simulink model "car_kin_test"  (R2018b)
settings: Solver=FixedStepAuto  StartTime=0.0  StopTime=50  FixedStep=0.05  RelTol=1e-3
libraries: simulink x2, autolibshared x1
settings Model: Creator=le'e'x'  LastModifiedBy=le'e'x'

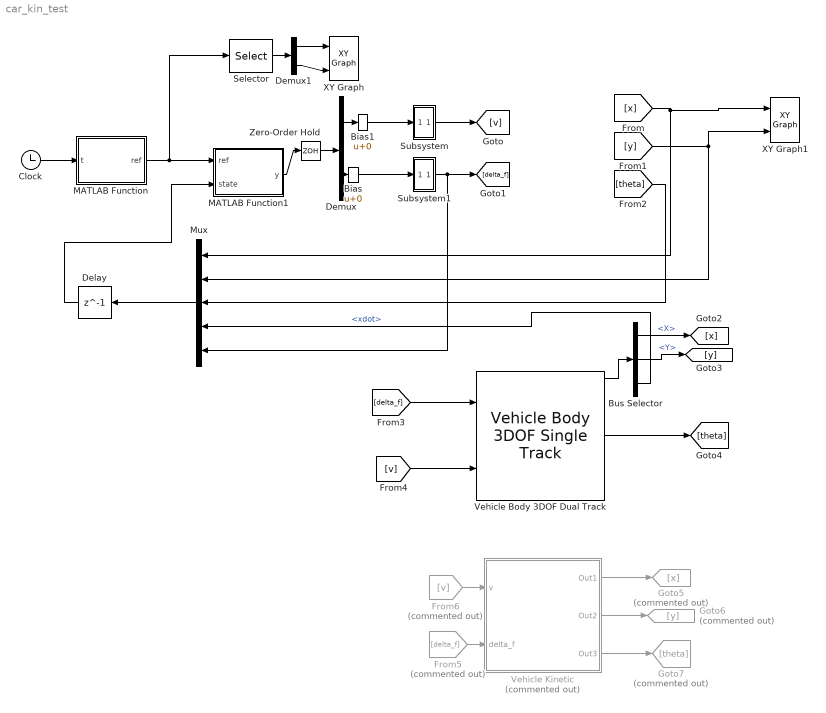
== system car_kin_test ==
  Bias : Bias
  Bias1 : Bias
  Bus Selector : BusSelector  OutputSignals=InertFrm.RearAxl.Disp.X,InertFrm.RearAxl.Disp.Y,BdyFrm.Cg.Vel.xdot
  Clock : Clock
  Delay : Delay  DelayLength=1  InitialCondition=[0 0 0 -0 0]
  Demux : Demux  Outputs=2
  Demux1 : Demux  Outputs=2
  From5 : From  Commented=on  GotoTag=delta_f
  From6 : From  Commented=on  GotoTag=v
  Goto5 : Goto  Commented=on  GotoTag=x
  Goto6 : Goto  Commented=on  GotoTag=y
  Goto7 : Goto  Commented=on  GotoTag=theta
  MATLAB Function : MATLAB Function  TreatAsAtomicUnit=on
  MATLAB Function1 : MATLAB Function  TreatAsAtomicUnit=on
  Mux : Mux  Inputs=5
  Selector : Selector  InputPortWidth=60  IndexOptions=Index vector (dialog)  Indices=[1 2]  OutputSizes=1
  Subsystem : Subsystem
  Subsystem1 : Subsystem
  Vehicle Body 3DOF Dual Track : autolibshared/Vehicle Body 3DOF Single Track  trackMode=Single (bicycle)  inputMode=External longitudinal velocity  frontSteerMode=on  rearSteerMode=off  windMode=off  muMode=off  extFMode=off  extMMode=off  aMode=2  NF=2  NR=2  m=2000  a=1.4  b=1.6  h=0.35  X_o=0  xdot_o=0  CalphaMode=off  sigmaMode=on  d=0  w=[1.4,1.4]  Cy_f=12e3  Cy_r=11e3  sigma_f=.1  sigma_r=.1  alpha_f_brk=[-.1 .1]  Cy_f_data=[-9e3 9e3]  alpha_r_brk=[-.1 .1]  Cy_r_data=[-9e3 9e3]  Y_o=0  ydot_o=0  Izz=4000  psi_o=0  r_o=0  Af=2  Cd=.3  Cl=.1  Cpm=.1  beta_w=[0:0.01:0.3]  Cs=[0:0.03:0.9]  Cym=[0:0.01:0.3]  Pabs=101325  Tair=273  g=9.81  mu=1  xdot_tol=.01  Fznom=5000  Fxtire_sat=7e4  Fytire_sat=7e4  longOff=0  latOff=0  vertOff=0
      settings: SourceProductName=Powertrain Blockset  SourceProductBaseCode=PW
  Vehicle Kinetic : Subsystem  Commented=on  AncestorBlock=my_library/Vehicle Kinetic  mask{x=0, y=0, fai=0, L=2.6}
      mask prompts: x "X_0"; y "Y_0"; fai "Phi_0"
      mask Display:
      | port_label('input',1,'v','texmode','on')
      | port_label('input',2,'\delta_f','texmode','on')
      | port_label('output',1,'x','texmode','on')
      | port_label('output',2,'y','texmode','on')
      | port_label('output',3,'\phi','texmode','on')
      | disp("Vehicle Kinetic")
  XY Graph : simulink/Sinks/XY Graph  xmin=-1  xmax=50  ymin=-1  ymax=2  st=-1
  XY Graph1 : simulink/Sinks/XY Graph  xmin=-1  xmax=50  ymin=-1  ymax=2  st=-1
  Zero-Order Hold : ZeroOrderHold  SampleTime=0.05
  wires:
  Clock/1 -> MATLAB Function/1(t)
  MATLAB Function/1(ref) -> Selector/1, MATLAB Function1/1(ref)
  MATLAB Function1/1(y) -> Zero-Order Hold/1
  Bias/1 -> Subsystem1/1(In1)
  Bias1/1 -> Subsystem/1(In1)
  [x] -> XY Graph1/1, Mux/1
  [y] -> XY Graph1/2, Mux/2
  [theta] -> Mux/3
  Mux/1 -> Delay/1
  Delay/1 -> MATLAB Function1/2(state)
  Zero-Order Hold/1 -> Demux/1
  Selector/1 -> Demux1/1
  Demux1/1 -> XY Graph/1
  Demux1/2 -> XY Graph/2
  Demux/2 -> Bias/1
  Demux/1 -> Bias1/1
  [delta_f] -> Vehicle Body 3DOF Dual Track/1
  [v] -> Vehicle Body 3DOF Dual Track/2
  Vehicle Body 3DOF Dual Track/1 -> Bus Selector/1
  Bus Selector/1 -> [x]  "<X>"
  Bus Selector/2 -> [y]  "<Y>"
  Vehicle Body 3DOF Dual Track/4 -> [theta]
  From5/1 -> Vehicle Kinetic/2(delta_f)
  From6/1 -> Vehicle Kinetic/1(v)
  Vehicle Kinetic/1(Out1) -> Goto5/1
  Vehicle Kinetic/3(Out3) -> Goto7/1
  Vehicle Kinetic/2(Out2) -> Goto6/1
  Bus Selector/3 -> Mux/4  "<xdot>"
  Subsystem/1(Out1) -> [v]
  Subsystem1/1(Out1) -> Mux/5, [delta_f]

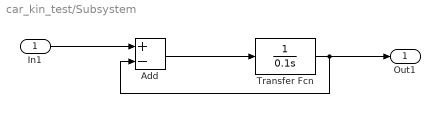
== system car_kin_test/Subsystem ==
  In1 : Inport
  Add : Sum  Inputs=+-
  Transfer Fcn : TransferFcn  Denominator=[0.1 0]
  Out1 : Outport
  wires:
  In1/1 -> Add/1
  Add/1 -> Transfer Fcn/1
  Transfer Fcn/1 -> Add/2, Out1/1

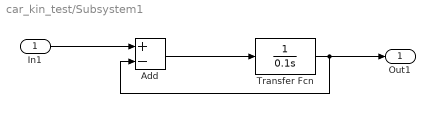
== system car_kin_test/Subsystem1 ==
  In1 : Inport
  Add : Sum  Inputs=+-
  Transfer Fcn : TransferFcn  Denominator=[0.1 0]
  Out1 : Outport
  wires:
  Transfer Fcn/1 -> Out1/1, Add/2
  In1/1 -> Add/1
  Add/1 -> Transfer Fcn/1

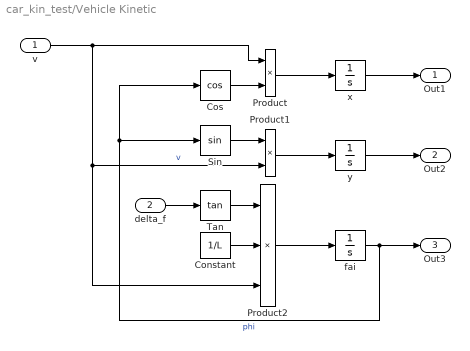
== system car_kin_test/Vehicle Kinetic ==
  v : Inport
  delta_f : Inport  Port=2
  Constant : Constant  Value=1/L
  Cos : Trigonometry  Operator=cos
  Product : Product
  Product1 : Product
  Product2 : Product  Inputs=3
  Sin : Trigonometry
  Tan : Trigonometry  Operator=tan
  fai : Integrator  InitialCondition=fai
  x : Integrator  InitialCondition=x
  y : Integrator  InitialCondition=y
  Out1 : Outport
  Out2 : Outport  Port=2
  Out3 : Outport  Port=3
  wires:
  x/1 -> Out1/1
  fai/1 -> Out3/1, Sin/1, Cos/1  "phi"
  Cos/1 -> Product/2
  v/1 -> Product2/3, Product1/2, Product/1  "v"
  Product/1 -> x/1
  Sin/1 -> Product1/1
  Product1/1 -> y/1
  y/1 -> Out2/1
  Tan/1 -> Product2/1
  Constant/1 -> Product2/2
  delta_f/1 -> Tan/1
  Product2/1 -> fai/1

== matlab function car_kin_test/MATLAB Function1 ==
  data: ref input; y output; state input
function y = myMPC(ref,state)
%#codegen
nc=2;
temp=zeros(2,1);
coder.extrinsic("mymex")
temp = mymex(ref,state);
y=temp;

== matlab function car_kin_test/MATLAB Function ==
  data: t input; ref output
function ref = fcn(t)
%#codegen
ts=0.05;
np=20;
dt=0:ts:(np-1)*ts;
ref=zeros(3*np,1);
for i=1:np
    ref((i-1)*3+1:i*3)=[dt(i)+t,1,0]';
end
